simulink subsystem "room"  (R2022b)
settings: Solver=VariableStepAuto  StartTime=0.0  StopTime=10.0  RelTol=1e-3
settings Model: Creator=aryan  LastModifiedBy=aryan

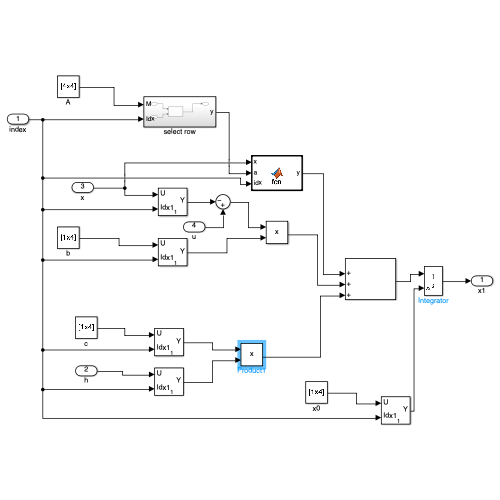
[thumbnail: Simulink's stored preview of the top-level diagram]
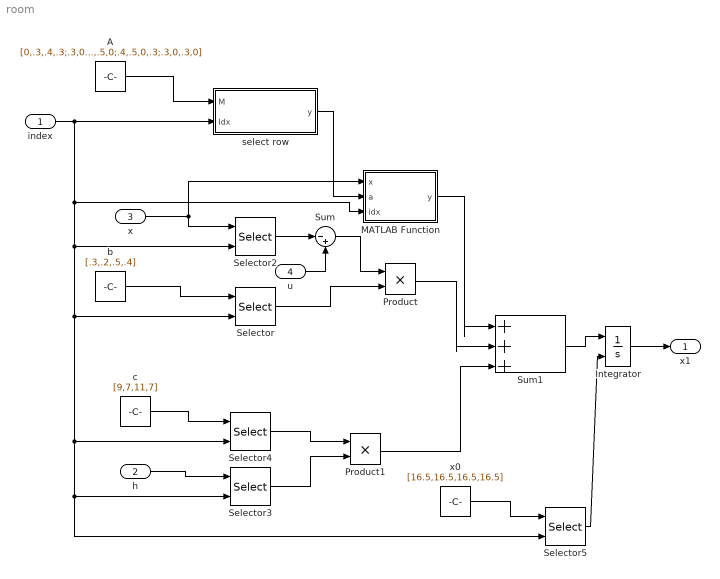
== system room ==
  index : Inport
  h : Inport  Port=2
  x : Inport  Port=3
  u : Inport  Port=4
  A : Constant  Value=[0,.3,.4,.3;.3,0,.5,0;.4,.5,0,.3;.3,0,.3,0]
  Integrator : Integrator  InitialConditionSource=external  InitialCondition=20
  MATLAB Function : MATLAB Function  TreatAsAtomicUnit=on
  Product : Product
  Product1 : Product
  Selector{,2..5} (5 alike) : Selector  InputPortWidth=4  IndexOptions=Index vector (port)  Indices=[1 3]  OutputSizes=1
  Sum : Sum  Inputs=|-+
  Sum1 : Sum  Inputs=|+++
  b : Constant  Value=[.3,.2,.5,.4]
  c : Constant  Value=[9,7,11,7]
  select row : Subsystem
  x0 : Constant  Value=[16.5,16.5,16.5,16.5]
  x1 : Outport
  wires:
  A/1 -> select row/1(M)
  select row/1(y) -> MATLAB Function/2(a)
  x0/1 -> Selector5/1
  MATLAB Function/1(y) -> Sum1/1
  u/1 -> Sum/2
  Integrator/1 -> x1/1
  Selector/1 -> Product/2
  Selector2/1 -> Sum/1
  Selector3/1 -> Product1/2
  b/1 -> Selector/1
  x/1 -> Selector2/1, MATLAB Function/1(x)
  index/1 -> select row/2(Idx), Selector2/2, Selector/2, Selector3/2, Selector5/2, Selector4/2, MATLAB Function/3(idx)
  c/1 -> Selector4/1
  Product1/1 -> Sum1/3
  Selector5/1 -> Integrator/2
  Sum/1 -> Product/1
  Sum1/1 -> Integrator/1
  Selector4/1 -> Product1/1
  h/1 -> Selector3/1
  Product/1 -> Sum1/2

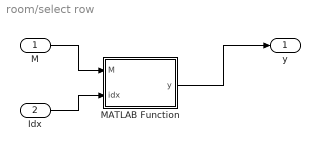
== system room/select row ==
  M : Inport
  Idx : Inport  Port=2
  MATLAB Function : MATLAB Function  TreatAsAtomicUnit=on
  y : Outport
  wires:
  M/1 -> MATLAB Function/1(M)
  Idx/1 -> MATLAB Function/2(idx)
  MATLAB Function/1(y) -> y/1

== matlab function room/select row/MATLAB Function ==
  data: M input; y output; idx input
function y = fcn(M,idx)

y = M(idx,:);

== matlab function room/MATLAB Function ==
  data: x input; y output; a input; idx input
function y = fcn(x,a,idx)
sum = 0;
for i = 1:4
    sum = sum + a(i) * (x(i)-x(idx));
end

y = sum;
